simulink model "gm_pulse_detector_v4_4"  (R2017b)
settings: Solver=FixedStepDiscrete  StartTime=0.0  StopTime=SimTime  RelTol=1e-3
undefined symbols (not defined in the file or in its folder): CorrFilter, RxSignal, threshold, WindowLen
libraries: dspsrcs4 x2, simulink x1, hdlsllib x1
settings Model: SimulationMode=accelerator  Creator=proso  LastModifiedBy=proso
settings DataIOCC: SaveOutput=off  SaveTime=off  ReturnWorkspaceOutputs=on
settings OptimizationCC: BlockReduction=off  ConditionallyExecuteInputs=off  DefaultParameterBehavior=Inlined
settings DebuggingCC: AlgebraicLoopMsg=error  InheritedTsInSrcMsg=none  SingleTaskRateTransMsg=error
settings HardwareCC: ProdBitPerPointer=32  ProdBitPerSizeT=32  ProdBitPerPtrDiffT=32  ProdLargestAtomicFloat=None  ProdIntDivRoundTo=Undefined  ProdEndianess=Unspecified  ProdWordSize=32  ProdHWDeviceType=ASIC/FPGA->ASIC/FPGA  TargetBitPerPointer=64  TargetBitPerSizeT=64  TargetBitPerPtrDiffT=64  TargetLongLongMode=on  TargetIntDivRoundTo=Zero  TargetEndianess=LittleEndian  TargetWordSize=64  TargetHWDeviceType=Custom Processor->MATLAB Host Computer  ProdEqTarget=off

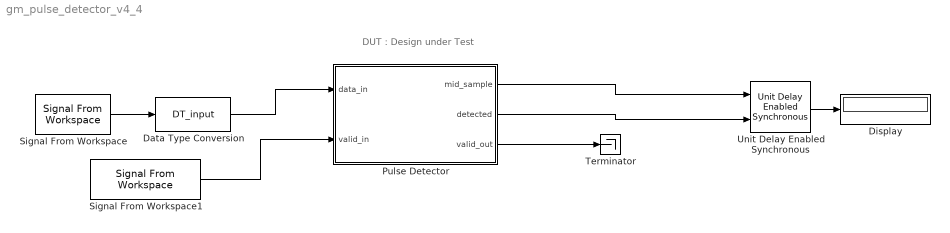
== system gm_pulse_detector_v4_4 ==
  note: DUT : Design under Test
  Data Type Conversion : DataTypeConversion  OutDataTypeStr=DT_input
  Display : Display
  Pulse Detector : Subsystem
  Signal From Workspace : dspsrcs4/Signal From Workspace  X=RxSignal  Ts=1  nsamps=1  OutputAfterFinalValue=Setting to zero  ignoreOrWarnInputAndFrameLengths=off  OutputFrames=off
  Signal From Workspace1 : dspsrcs4/Signal From Workspace  X=true(size(RxSignal))  Ts=1  nsamps=1  OutputAfterFinalValue=Setting to zero  ignoreOrWarnInputAndFrameLengths=off  OutputFrames=off
  Terminator : Terminator
  Unit Delay Enabled Synchronous : hdlsllib/Discrete/Unit Delay Enabled Synchronous  InitialCondition=0.0  SampleTime=-1
      settings: SourceProductName=HDL Coder  SourceProductBaseCode=HD
  wires:
  Data Type Conversion/1 -> Pulse Detector/1(data_in)
  Signal From Workspace/1 -> Data Type Conversion/1
  Pulse Detector/3(valid_out) -> Terminator/1
  Signal From Workspace1/1 -> Pulse Detector/2(valid_in)
  Pulse Detector/2(detected) -> Unit Delay Enabled Synchronous/2
  Pulse Detector/1(mid_sample) -> Unit Delay Enabled Synchronous/1
  Unit Delay Enabled Synchronous/1 -> Display/1

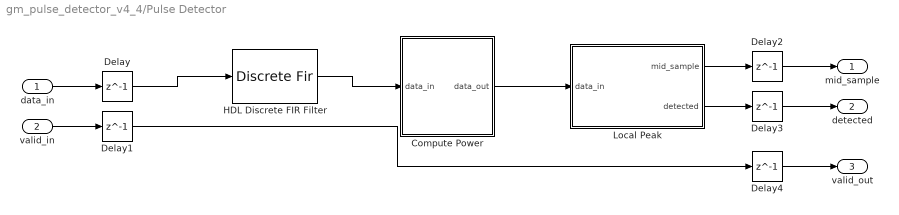
== system gm_pulse_detector_v4_4/Pulse Detector ==
  data_in : Inport  OutDataTypeStr=fixdt(1, 16, 14)  SampleTime=1
      settings: SignalType=complex
  valid_in : Inport  Port=2  OutDataTypeStr=boolean  SampleTime=1
  Compute Power : Subsystem
  Delay{,1..4} (5 alike) : Delay  DelayLength=1
  HDL Discrete FIR Filter : DiscreteFir  FilterStructure=Direct form transposed  Coefficients=CorrFilter  CoefDataTypeStr=DT_coeff
  Local Peak : Subsystem
  mid_sample : Outport
  detected : Outport  Port=2
  valid_out : Outport  Port=3
  wires:
  data_in/1 -> Delay/1
  valid_in/1 -> Delay1/1
  Compute Power/1(data_out) -> Local Peak/1(data_in)
  Delay/1 -> HDL Discrete FIR Filter/1
  Delay1/1 -> Delay4/1
  Delay2/1 -> mid_sample/1
  Delay3/1 -> detected/1
  Delay4/1 -> valid_out/1
  HDL Discrete FIR Filter/1 -> Compute Power/1(data_in)
  Local Peak/1(mid_sample) -> Delay2/1
  Local Peak/2(detected) -> Delay3/1

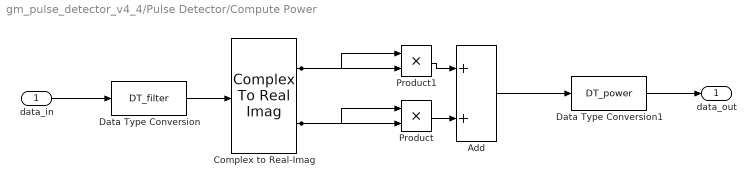
== system gm_pulse_detector_v4_4/Pulse Detector/Compute Power ==
  data_in : Inport  SampleTime=1
  Add : Sum
  Complex to Real-Imag : ComplexToRealImag
  Data Type Conversion : DataTypeConversion  OutDataTypeStr=DT_filter
  Data Type Conversion1 : DataTypeConversion  OutDataTypeStr=DT_power
  Product : Product
  Product1 : Product
  data_out : Outport
  wires:
  data_in/1 -> Data Type Conversion/1
  Add/1 -> Data Type Conversion1/1
  Complex to Real-Imag/1 -> Product1/2, Product1/1
  Complex to Real-Imag/2 -> Product/2, Product/1
  Data Type Conversion/1 -> Complex to Real-Imag/1
  Data Type Conversion1/1 -> data_out/1
  Product/1 -> Add/2
  Product1/1 -> Add/1

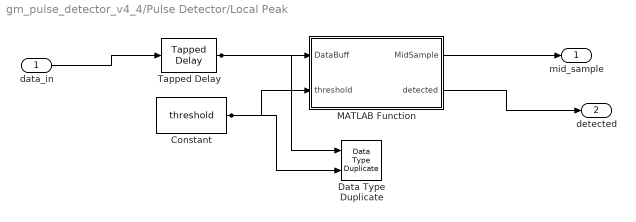
== system gm_pulse_detector_v4_4/Pulse Detector/Local Peak ==
  data_in : Inport  SampleTime=1
  Constant : Constant  Value=threshold  OutDataTypeStr=Inherit: Inherit via back propagation  SampleTime=-1
  Data Type Duplicate : DataTypeDuplicate
  MATLAB Function : Subsystem
  Tapped Delay : simulink/Discrete/Tapped Delay  vinit=0.0  samptime=-1  NumDelays=WindowLen  DelayOrder=Oldest  includeCurrent=off
  mid_sample : Outport
  detected : Outport  Port=2
  wires:
  data_in/1 -> Tapped Delay/1
  Constant/1 -> Data Type Duplicate/2, MATLAB Function/2(threshold)
  MATLAB Function/1(MidSample) -> mid_sample/1
  MATLAB Function/2(detected) -> detected/1
  Tapped Delay/1 -> Data Type Duplicate/1, MATLAB Function/1(DataBuff)

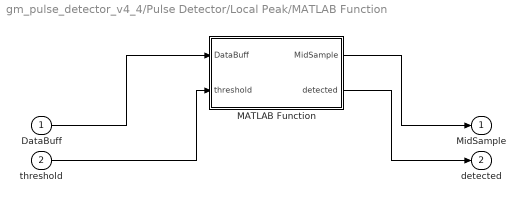
== system gm_pulse_detector_v4_4/Pulse Detector/Local Peak/MATLAB Function ==
  DataBuff : Inport  PortDimensions=11  SampleTime=1
  threshold : Inport  Port=2  SampleTime=1
  MATLAB Function : MATLAB Function  TreatAsAtomicUnit=on
  MidSample : Outport
  detected : Outport  Port=2
  wires:
  DataBuff/1 -> MATLAB Function/1(DataBuff)
  threshold/1 -> MATLAB Function/2(threshold)
  MATLAB Function/1(MidSample) -> MidSample/1
  MATLAB Function/2(detected) -> detected/1

== matlab function gm_pulse_detector_v4_4/Pulse Detector/Local Peak/MATLAB Function/MATLAB Function ==
  settings: fimath=fimath('RoundingMethod', 'Floor','OverflowAction', 'Wrap','ProductMode', 'FullPrecision', 'SumMode', 'FullPrecision')
  data: MidSample output; DataBuff input; threshold input; detected output; WindowLen parameter
function [MidSample,detected] = fcn(DataBuff,threshold, WindowLen)
   
MidIdx = ceil(WindowLen/2);
% Sliding window operation

% Compare each value in the window to the middle sample via subtraction
MidSample = DataBuff(MidIdx);
CompareOut = DataBuff - MidSample; % this is a vector

% if all values in the result are negative and the middle sample is
% greater than a threshold, it is a local max
if all(CompareOut <= 0) && (MidSample > threshold)
    detected = true;
else 
    detected = false;
end
